simulink model "bci_1d_horizontal_control_current_system_adaptivev2"  (R2013a)
settings: Solver=ode3  SolverMode=SingleTasking  StartTime=0.0  StopTime=inf  RelTol=1e-3
InitFcn:
  | clc
  | clear
  | close all
  | 
  | gnom = 70;
  | gmax = 80;
  | RunTrials = 2;
  | 
  | 
  | 
  | 
  | tic
  | fs = 125;
  | BufferLength = 12;
  | %12 previous trials
  | Nsd = 13;
  | phase = 1;%horizontal phase
  | dim = 1;
  | all = true;
  | first_session = true;
  | count = 0;
  |  %online feature update
  | 
  | std_dx =1;
  | mean_dx =0;
  | beta_x = [1;1;-1;-1];
  | std_prev = std_dx;
  | 
  | if std_dx < gnom
  |     std_test = gnom*std_dx/std_prev;
  |     if std_test < gnom
  |         b = gnom/std_dx;
  |     elseif (std_test>=gnom) &&(std_test <=gmax)
  |         b = gnom/std_prev;
  |     else
  |        b = gmax/std_dx;
  |     end
  | elseif (std_dx >= gnom) && (std_dx <= gmax)
  |     b = 1;
  | else
  |     b = gmax/std_dx;
  | end
  | 
  | %update sumilink model
  | val = [beta_x' mean_dx 1/b];
  | valString = strcat('[',num2str(val),']');
  | set_param('bci_1d_horizontal_control_current_system_adaptivev2/model_parameters','Value',valString);
  | toc
  | 
  | %resume simulation
  | set_param('bci_1d_horizontal_control_current_system_adaptivev2','SimulationCommand','continue');
  | disp('... Resume simulation...')
StopFcn:
  | %BackUp data first
  | time = clock();
  | date = [num2str(time(3)),'_',num2str(time(2)),'_',num2str(time(1))];
  | date = [date ,'_',num2str(time(4)),'h',num2str(time(5))];
  | 
  | save(['today_simout_backup','_',date,'.mat'])
model workspace (MAT data in the model file):
  local_ip = 2130706433
  local_port = 50224
  host_ip = 2130706433
  host_port = 50223
  serial_number = 'NB-2014.07.69'
  sample_rate = 250
  num_samples = 8
  num_en_channels = 32
  en_add_channels = 5
  cfg_native : struct (value not decoded)
undefined symbols (not defined in the file): NB
libraries: dspspect3 x4, dspnetwork x3, simulink x1, gNautilusLib x1
PauseFcn:
  | tic
  | fs = 125;
  | BufferLength = 12;%12 previous trials
  | Nsd = 13;
  | phase = 1;%horizontal phase
  | dim = 1;
  | all = true;
  | first_session = true;
  | count = count + 1;
  | 
  | %get training sets
  | [F,D,Fy,Dy,Fcell_x,Fcell_y,targets] = getTrainingSetsMLR(sim_out,BufferLength,phase,dim,Nsd,all);
  | 
  | %online feature update
  | c = str2num(get_param('bci_1d_horizontal_control_current_system_adaptivev2/model_parameters','Value'));
  | bprev = c(end);
  | mean_dx = c(end-1);
  | beta_x = c(1:(end-2))';
  | tid = targets{end};%target id
  | tcoords = bci_get_target_coord(tid,1);
  | 
  | disp('...LMS update ....')
  | 
  | %gain and mean adjsustment
  | if (mod(count,RunTrials) == 0) && (count ~= 0)
  | Dx = mlr_regressor2(beta_x,F);
  | [mean_dx,std_dx] = zscore_norm(Dx);
  | 
  | if std_dx < gnom
  |     std_test = gnom*std_dx/std_prev;
  |     if std_test < gnom
  |         b = gnom/std_dx;
  |     elseif (std_test>=gnom) &&(std_test <=gmax)
  |         b = gnom/std_prev;
  |     else
  |        b = gmax/std_dx;
  |     end
  | elseif (std_dx >= gnom) && (std_dx <= gmax)
  |     b = 1;
  | else
  |     b = gmax/std_dx;
  | end
  |   std_prev = std_dx;
  | disp('---mean --gain update---')
  | mean_dx
  | b
  | std_dx
  | end
  | 
  | if ~isnan(mean_dx)
  | %update sumilink model
  | val = [beta_x' mean_dx 1/b];
  | valString = strcat('[',num2str(val),']');
  | set_param('bci_1d_horizontal_control_current_system_adaptivev2/model_parameters','Value',valString);
  | end
  | toc
  | 
  | set_param('bci_1d_horizontal_control_current_system_adaptivev2/model_parameters','Value',valString);
  | 
  | %resume simulation
  | set_param('bci_1d_horizontal_control_current_system_adaptivev2','SimulationCommand','continue');
  | disp('... Resume simulation...')
settings Model: ExtModeTrigDuration=2  Creator=Yves Matanga  LastModifiedBy=Yves Matanga
settings OptimizationCC: OptimizeModelRefInitCode=on  LifeSpan=1
settings DebuggingCC: SolverPrmCheckMsg=none  StrictBusMsg=Warning
settings HardwareCC: ProdBitPerInt=16  ProdBitPerPointer=8  ProdIntDivRoundTo=Zero  ProdEndianess=LittleEndian  ProdWordSize=8  ProdHWDeviceType=Atmel->AVR
settings RTWCC: SystemTargetFile=realtime.tlc  GenerateMakefile=off  TemplateMakefile=realtime.tmf  Description=Run on Target Hardware  RTWVerbose=off  ProcessScript=realtime_make_rtw_hook
settings STFCustomTargetCC: TargetLibSuffix=.a  GenerateSampleERTMain=on  ERTCustomFileBanners=on  SupportNonInlinedSFcns=off  SupportVariableSizeSignals=on  MATLABClassNameForMDSCustomization=Simulink.SoftwareTarget.ERTCustomization  SystemTargetFile=realtime.tlc
settings ERTTargetCC: ParMdlRefBuildCompliant=off  CompOptLevelCompliant=off  ConcurrentExecutionCompliant=off  CombineOutputUpdateFcns=off  ERTFirstTimeCompliant=off  SupportContinuousTime=on  SupportVariableSizeSignals=on  ModelStepFunctionPrototypeControlCompliant=off  CPPClassGenCompliant=off  ExtMode=on  ExtModeTransport=3  ExtModeMexFile=ext_serial_win32_comm  ExtModeMexArgs=0 1 9600  ERTSrcFileBannerTemplate=realtime_code_template.cgt  ERTHdrFileBannerTemplate=realtime_code_template.cgt  ERTDataSrcFileTemplate=realtime_code_template.cgt  ERTDataHdrFileTemplate=realtime_code_template.cgt  ERTCustomFileTemplate=realtime_file_process.tlc

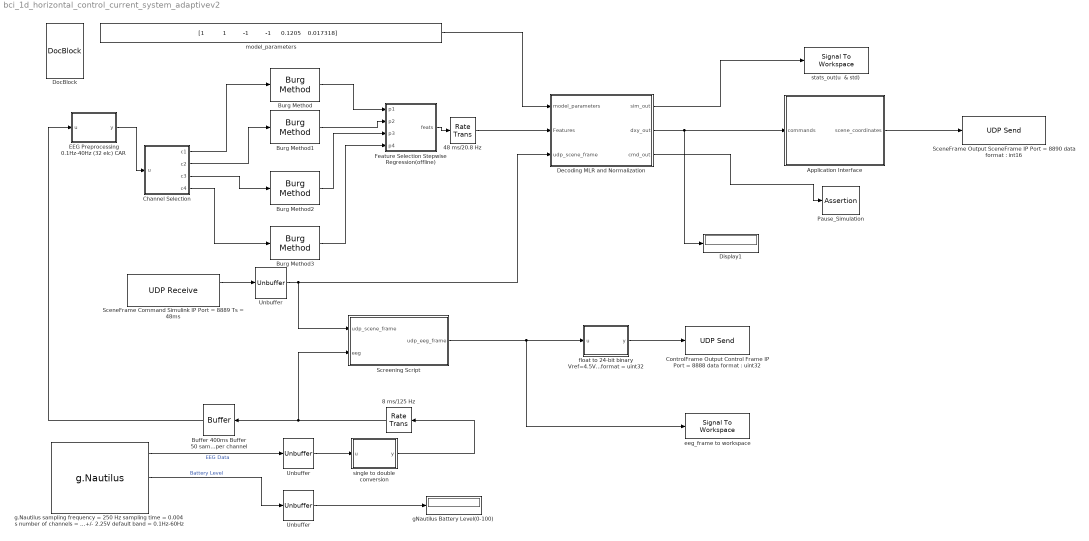
== system bci_1d_horizontal_control_current_system_adaptivev2 ==
  " 48 ms/20.8 Hz " : RateTransition  OutPortSampleTime=0.048
  8 ms/125 Hz : RateTransition  OutPortSampleTime=0.008
  Application Interface : MATLAB Function  TreatAsAtomicUnit=on  SystemSampleTime=0.048
  Buffer 400ms Buffer 50 samples per channel : Buffer  N=50  V=49  TreatMby1Signals=One channel
  Burg Method{,1..3} (4 alike) : dspspect3/Burg Method  inheritOrd=off  ord=16  inheritFFT=off  fftsize=1024  inheritTs=on  Ts=1
  Channel Selection : MATLAB Function  TreatAsAtomicUnit=on  SystemSampleTime=0.008
  "ControlFrame Output Control Frame IP Port = 8888 data format : uint32" : dspnetwork/UDP Send  remoteURL='127.0.0.1'  remotePort=8888  localURL='0.0.0.0'  localPortSource=Automatically determine  localPort=-1  sampletime=-1  separateLengthPort=0
  Decoding MLR and Normalization : MATLAB Function  TreatAsAtomicUnit=on  SystemSampleTime=0.048
  Display1 : Display
  DocBlock : simulink/Model-Wide Utilities/DocBlock  DocumentType=Text
      content=|
      | The Above platform is for EEG capturing a
      | and samping of screening imagery .
      |
      | A JAVA GUI is running aside this simulink and communicate
      | via UDP protocol
      |
      | Once the Screening start ,the Java scene GUI send a start
      | command to the simulink model (ASCII for '1' ) which
      | will trigger a sampling signal to 1
      |
      | Once the Screening stopped ,the Java GUI will send a stop command
      | to the simulink model (ASCII for '2') which will trigger
      | a sampling signal to 2
      |
      | else it iso 0
      |
      | the sampling signal will help extract the eeg signals of the
      | user motor imagery ,hence
      |
      | the interval between a start (1) and a stop (2) is
      | basically "a single trial eeg imagery"
      |
      | all the eeg signals will be transferred at all time to the java
      | application which save into a database for furhter recovery.
      |
      | Note that all blocks must have the sampling time as dictated by the EEG source
      | T = 0.004s (250Hz)
      |
      | ---------------------------------------------------------------------------------------------------------
      | UPDATES :
      |
      | (*) Target Number Reception Included (From JAVA SceneControlPanel)
      | (*) Training From N (10 = default) previous trials datasets very well now(with variable size)
      |
      | Problems :
      |
      | (*) How To Update Previous BCI weights to the current one
      |     Make Sure You Save Them in The Database for later use
      | (*) Output Normalization Must not be based upon the previous feature only because (they can be an error in the
      |     previous trial)
      | (*) Is There A Real Need for input Normalization ????
      | (*) How To Take Care of Nan in Features because they disrupt the feature set selection process
      |
      | Solution :
      |
      | (*) May be you can discard trials with Nan Features  ---> Just Make Sure To Count How Many
      | They are to see if it is really relevant
  EEG Preprocessing 0.1Hz-40Hz (32 elc) CAR : MATLAB Function  TreatAsAtomicUnit=on  SystemSampleTime=0.008
  Feature Selection Stepwise Regression(offline) : MATLAB Function  TreatAsAtomicUnit=on  SystemSampleTime=0.008
  Pause_Simulation : Assertion  AssertionFailFcn=|  StopWhenAssertionFail=off  SampleTime=0.048
      | set_param(bdroot,'SimulationCommand','pause'),
      | disp(sprintf('\nSimulation paused.'))
  SceneFrame Command Simulink IP Port = 8889 Ts = 48ms : dspnetwork/UDP Receive  localURL='0.0.0.0'  localPort=8889  remoteURL='127.0.0.1'  remotePort=-1  recvBufferSize=8192  dims=255  signalDatatype=uint8  isVarSize=off  showBlockingTime=off  blockingTime=0  sampletime=0.048
  "SceneFrame Output SceneFrame IP Port = 8890 data format : int16" : dspnetwork/UDP Send  remoteURL='127.0.0.1'  remotePort=8890  localURL='0.0.0.0'  localPortSource=Automatically determine  localPort=-1  sampletime=-1  separateLengthPort=0
  Screening Script : MATLAB Function  TreatAsAtomicUnit=on  SystemSampleTime=0.008
  Unbuffer : Unbuffer  SampleBasedProcessing=Same as frame based
  "Unbuffer " : Unbuffer  SampleBasedProcessing=Same as frame based
  "Unbuffer   " : Unbuffer  SampleBasedProcessing=Same as frame based
  eeg_frame to workspace : SignalToWorkspace  VariableName=eeg_frame
      settings: CopyFcn=dspblkcopystw(gcbh);
  float to 24-bit binary Vref=4.5V(in uV) Mean = 2.25V data format = uint32 : MATLAB Function  TreatAsAtomicUnit=on  SystemSampleTime=0.008
  "g.Nautilus sampling frequency = 250 Hz sampling time = 0.004 s number of channels = 32 resolution = 24 Bit output = float32 unit = uV dynamic range = +/- 2.25V default band = 0.1Hz-60Hz " : gNautilusLib/g.Nautilus  Tag=g.Nautilus  Description=Operates a g.Nautilus device and provides acquired data on its outputs.  sample_rate=250  local_ip=2130706433  local_port=50224  host_ip=2130706433  host_port=50223  serial_number=NB-2014.07.69  num_samples=8  num_en_channels=32  add_channels=5
  gNautilus Battery Level(0-100) : Display
  model_parameters : Constant  Value="[1           1          -1          -1      0.1205    0.017318]"  SampleTime=-1
  single to double conversion : MATLAB Function  TreatAsAtomicUnit=on  SystemSampleTime=0.004
  stats_out(u  & std) : SignalToWorkspace  VariableName=sim_out
      settings: CopyFcn=dspblkcopystw(gcbh);
  wires:
  "g.Nautilus sampling frequency = 250 Hz sampling time = 0.004 s number of channels = 32 resolution = 24 Bit output = float32 unit = uV dynamic range = +/- 2.25V default band = 0.1Hz-60Hz "/1 -> Unbuffer/1  "EEG Data"
  Unbuffer/1 -> single to double conversion/1(u)
  SceneFrame Command Simulink IP Port = 8889 Ts = 48ms/1 -> "Unbuffer "/1
  8 ms/125 Hz/1 -> Buffer 400ms Buffer 50 samples per channel/1, Screening Script/2(eeg)
  float to 24-bit binary Vref=4.5V(in uV) Mean = 2.25V data format = uint32/1(y) -> "ControlFrame Output Control Frame IP Port = 8888 data format : uint32"/1
  single to double conversion/1(y) -> 8 ms/125 Hz/1
  Screening Script/1(udp_eeg_frame) -> float to 24-bit binary Vref=4.5V(in uV) Mean = 2.25V data format = uint32/1(u), eeg_frame to workspace/1
  EEG Preprocessing 0.1Hz-40Hz (32 elc) CAR/1(y) -> Channel Selection/1(u)
  "Unbuffer   "/1 -> gNautilus Battery Level(0-100)/1
  "g.Nautilus sampling frequency = 250 Hz sampling time = 0.004 s number of channels = 32 resolution = 24 Bit output = float32 unit = uV dynamic range = +/- 2.25V default band = 0.1Hz-60Hz "/2 -> "Unbuffer   "/1  "Battery Level"
  Buffer 400ms Buffer 50 samples per channel/1 -> EEG Preprocessing 0.1Hz-40Hz (32 elc) CAR/1(u)
  Feature Selection Stepwise Regression(offline)/1(feats) -> " 48 ms/20.8 Hz "/1
  " 48 ms/20.8 Hz "/1 -> Decoding MLR and Normalization/2(Features)
  model_parameters/1 -> Decoding MLR and Normalization/1(model_parameters)
  Decoding MLR and Normalization/3(cmd_out) -> Pause_Simulation/1
  Decoding MLR and Normalization/1(sim_out) -> stats_out(u  & std)/1
  "Unbuffer "/1 -> Decoding MLR and Normalization/3(udp_scene_frame), Screening Script/1(udp_scene_frame)
  Application Interface/1(scene_coordinates) -> "SceneFrame Output SceneFrame IP Port = 8890 data format : int16"/1
  Decoding MLR and Normalization/2(dxy_out) -> Display1/1, Application Interface/1(commands)
  Channel Selection/1(c1) -> Burg Method/1
  Burg Method/1 -> Feature Selection Stepwise Regression(offline)/1(p1)
  Channel Selection/2(c2) -> Burg Method1/1
  Burg Method1/1 -> Feature Selection Stepwise Regression(offline)/2(p2)
  Channel Selection/3(c3) -> Burg Method2/1
  Channel Selection/4(c4) -> Burg Method3/1
  Burg Method3/1 -> Feature Selection Stepwise Regression(offline)/4(p4)
  Burg Method2/1 -> Feature Selection Stepwise Regression(offline)/3(p3)

== matlab function bci_1d_horizontal_control_current_system_adaptivev2/single to double conversion ==
  data: u input; y output
function y = fcn(u)
%#codegen
y = double(u);

== matlab function bci_1d_horizontal_control_current_system_adaptivev2/Screening Script ==
  data: udp_scene_frame input; eeg input; udp_eeg_frame output
function udp_eeg_frame  = fcn( udp_scene_frame,eeg)
%#codegen
 if udp_scene_frame == uint8('1') %START in ASCII
     udp_eeg_frame = [eeg 1];%timing frame = 1
 elseif udp_scene_frame == uint8('2') %STOP
     udp_eeg_frame = [eeg 2];%timing frame = 2
 else
     udp_eeg_frame = [eeg 0];%timing frame = 0
 end
 
 %the purpose of this function to 
 %save the  eeg signals sampled with the start
 %and stop of every trial%

== matlab function bci_1d_horizontal_control_current_system_adaptivev2/EEG Preprocessing 0.1Hz-40Hz (32 elc) CAR ==
  data: u input; y output
function y = fcn(u)
%Input EEG (0.1Hz - 60Hz) with 50Hz Notch
%Preprocessing Stage (0.1Hz - 40Hz) Signal 
%fHigh = 40;% 40Hz
%fs = 250;%250Hz
%order = 5 ;% Filter Order
%[bw,aw] = butter(order,[fHigh]/(fs/2));%Butterworth filter
%yf = filter(bw,aw,u);%filtered ( < 40Hz)
%y = eegHjorthSL(u);%Surface Laplacian 
%(Large Laplacian : Must Be Small Laplacian as you're using 32 electrodes)
y = eegCarf(u);%Common Average

== matlab function bci_1d_horizontal_control_current_system_adaptivev2/float to 24-bit binary Vref=4.5V(in uV) Mean = 2.25V data format = uint32 ==
  data: u input; y output
function y = fcn(u)
 eeg_frame = u(1:32);
 %convert to 24 bit binary
 bin = uint32((eeg_frame + 2.25e6)*(2^24-1)/(4.5e6));
y = [bin uint32(u(33))]; %Select All Channels

== matlab function bci_1d_horizontal_control_current_system_adaptivev2/Channel Selection ==
  data: c1 output; c2 output; u input; c3 output; c4 output
function [c1,c2,c3,c4] = fcn(u)
%#codegen

%channel lookup table
% 1 --  FP1                      % 17 --  C4
% 2 --  FP2                      % 18 --  T8
% 3 --  AF3                      % 19 --  CP5
% 4 --  AF4                      % 20 --  CP1
% 5 --  F7                       % 21 --  CP2
% 6 --  F3                       % 22 --  CP6
% 7 --  FZ                       % 23 --  P7 
% 8 --  F4                       % 24 --  P3
% 9 --  F8                       % 25 --  PZ
% 10 -- FC5                      % 26 --  P4
% 11 -- FC1                      % 27 --  P8
% 12 -- FC2                      % 28 --  PO7
% 13 -- FC6                      % 29 --  PO3
% 14 -- T7                       % 30 --  PO4
% 15 -- C3                       % 31 --  PO8
% 16 -- CZ                       % 32 --  OZ

%Ch = [15 17];
%c1 = u(:,21); %cp2
%c2 = u(:,16); % cz
%c3 = u(:,15); %c3
%c4 = u(:,19); % cp5

c1 = u(:,21); %cp2
c2 = u(:,16); % cz
c3 = u(:,25); %c3
c4 = u(:,17); % cp5

== matlab function bci_1d_horizontal_control_current_system_adaptivev2/Application Interface ==
  data: commands input; scene_coordinates output
function scene_coordinates = fcn(commands)
%#codegen
% persistent dy;
% step = 1;%pixel setp
% screenHeight = 1018;
% if isempty(dy)
%     dy = -3*screenHeight/8;
% end
%sending daa via UDP
scene_coordinates = [int16(commands(1)) int16(commands(2))];
%dy = dy + step;%cursor moving up in y direction...

== matlab function bci_1d_horizontal_control_current_system_adaptivev2/Feature Selection Stepwise Regression(offline) ==
  data: p1 input; feats output; p2 input; p3 input; p4 input
function feats = fcn(p1,p2,p3,p4)
%features selection
fs = 125;
df = 3;%3Hz wide band  3Hz band 



freqs1 = [26];%24.5Hz - 27.5Hz centré sur 26Hz 
freqs2 = [29];
freqs3 = [8];
freqs4 = [23];



feats1 = bci_freq2band(sqrt(p1),freqs1,df,fs);
feats2 = bci_freq2band(sqrt(p2),freqs2,df,fs);
feats3 = bci_freq2band(sqrt(p3),freqs3,df,fs);
feats4 = bci_freq2band(sqrt(p4),freqs4,df,fs);

 feats = [feats1 feats2 feats3 feats4];

== matlab function bci_1d_horizontal_control_current_system_adaptivev2/Decoding MLR and Normalization ==
  data: sim_out output; dxy_out output; cmd_out output; model_parameters input; Features input; udp_scene_frame input

function [sim_out,dxy_out,cmd_out] = fcn(model_parameters,Features,udp_scene_frame)
%variable declarations
persistent target_id;%position of target in scenario
persistent dy;
persistent cmd;
persistent gain;
% persistent check;
% persistent std_d0;
persistent SUM_X;
persistent SUM_Y;
persistent SUM;



%gain = 13;%15*screenHeight*3/(8*Nht);%with a slow moving cursor
mean_dx = model_parameters(end-1); 
std_dx = model_parameters(end);    
if (isempty(target_id))%by deault consider target 1
   target_id=1;
   dy =  0;%3
   cmd = 1;
   gain =  1;%
%    check = mean_dx;
%    std_d0 = 48;
end
dxy = zeros(1,2);
dxy_raw = zeros(1,2);
%trainging time
if ~isempty(find(udp_scene_frame==uint8('1')))%start of paradigm       
    sync = 1;    
    cmd = 1;
elseif ~isempty(find(udp_scene_frame==uint8('2'))) %STOP PRACTICE       
    sync = 2; 
    cmd = 0;%pause simulation to retrain
elseif ~isempty(find((udp_scene_frame >=uint8('3')) & ...
        (udp_scene_frame <=uint8('6')) ))%target number received
    sync = 0;
    target_id= double(udp_scene_frame(1)-48-2);    
    cmd = 1;
else
    sync = 0;%for timing of data
    cmd = 1;
end

%real time regression
beta_x = model_parameters(1:end-2);

%avoiding Nan
Fn = zeros(1,size(Features,2));
if sum(isnan(Features)) == 0
    Fn = Features;
    gain = 1;
else
    Fn = zeros(1,length(Features));
    gain = 0;
end
dxy_raw(1) =  mlr_regressor2(beta_x,Fn); %c
dxy_raw(2) = dy;
%output normalization
dxy(1) = 0.1*gain*zscore(dxy_raw(1),mean_dx,std_dx);%
dxy(2) = dxy_raw(2);
%append sync to facilitate data removal


dxy_out = dxy;


sim_out = [beta_x' mean_dx std_dx dxy dxy_raw Fn target_id sync];
%simulation commands
cmd_out = cmd;%
